simulink model "relay_model_gea_2017a"  (R2019b)
settings: Solver=VariableStepAuto  StartTime=0.0  StopTime=Tsim  RelTol=1e-6
values from neighbouring files (symbols this model uses):
  a1 = x(3)    [relaysim.m]
  a2 = x(2)    [relaysim.m]
  den = sym2poly((s+1)*(0.1*s+1)*(0.01*s+1))    [get_function.m]
  K = x(1)    [relaysim.m]
  num = 1    [get_function.m]
  Td = x(4)    [relaysim.m]
undefined symbols (not defined in the file or in its folder): rd, ri, rp, step_in, Tds
libraries: simulink x1
settings Model: Creator=export08  LastModifiedBy=adrian
settings DataIOCC: ReturnWorkspaceOutputs=off
settings DebuggingCC: ArithmeticOperatorsInVariantConditions=warning
settings SFSimCC: SimUseLocalCustomCode=off  CustomCodeUndefinedFunction=UseInterfaceOnly
settings RTWCC: RTWUseLocalCustomCode=off
settings CodeAppCC: StateflowObjectComments=on

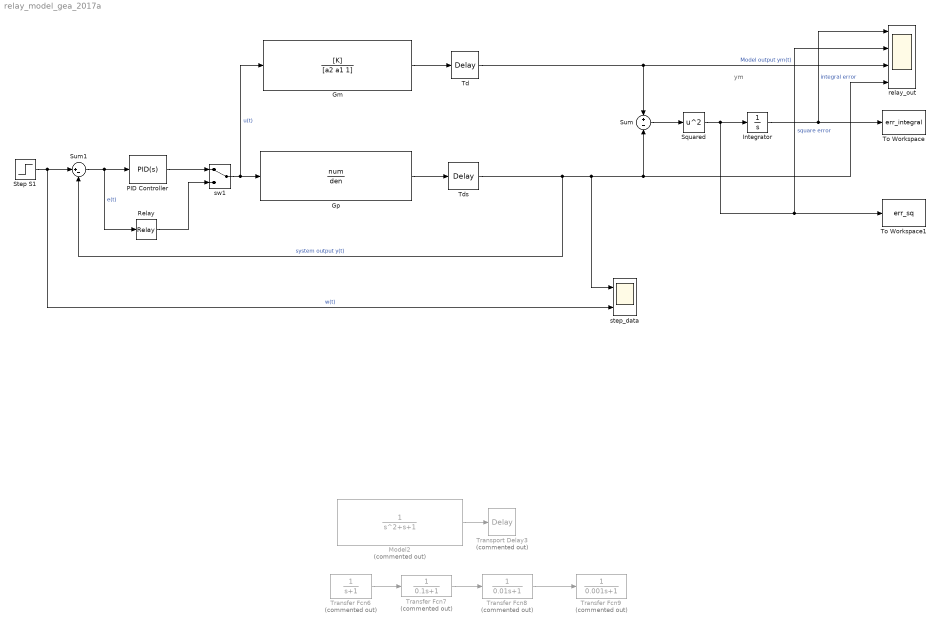
== system relay_model_gea_2017a ==
  note: ym
  Gm : TransferFcn  Numerator=[K]  Denominator=[a2 a1 1]
  Gp : TransferFcn  Numerator=num  Denominator=den
  Integrator : Integrator
  Model2 : TransferFcn  Commented=on  Numerator=1  Denominator=[1 1 1]
  PID Controller : simulink/Continuous/PID Controller  Controller=PID  Form=Parallel  TimeDomain=Continuous-time  SampleTime=-1  IntegratorMethod=Forward Euler  FilterMethod=Forward Euler  ControllerParametersSource=internal  P=rp  I=ri  D=rd  UseFilter=on  N=100  TunerSelectOption=Transfer Function Based (PID Tuner App)  InitialConditionSource=internal  InitialConditionForIntegrator=0  InitialConditionForFilter=0  DifferentiatorICPrevScaledInput=0  ExternalReset=none  TrackingMode=off  Kt=1  LimitOutput=off  UpperSaturationLimit=inf  LowerSaturationLimit=-inf  LinearizeAsGain=on  AntiWindupMode=none  Kb=1  POutMin=[]  POutMax=[]  IOutMin=[]  IOutMax=[]  DOutMin=[]  DOutMax=[]  NOutMin=[]  NOutMax=[]  SumOutMin=[]  SumOutMax=[]  SaturationOutMin=[]  SaturationOutMax=[]  PParamMin=[]  PParamMax=[]  IParamMin=[]  IParamMax=[]  DParamMin=[]  DParamMax=[]  NParamMin=[]  NParamMax=[]  KbParamMin=[]  KbParamMax=[]  KtParamMin=[]  KtParamMax=[]  KbOutMin=[]  KbOutMax=[]  KtOutMin=[]  KtOutMax=[]  IntegratorOutMin=[]  IntegratorOutMax=[]  FilterOutMin=[]  FilterOutMax=[]  SumI1OutMin=[]  SumI1OutMax=[]  SumI2OutMin=[]  SumI2OutMax=[]  SumI3OutMin=[]  SumI3OutMax=[]  SumI4OutMin=[]  SumI4OutMax=[]  SumDOutMin=[]  SumDOutMax=[]  DifferentiatorOutMin=[]  DifferentiatorOutMax=[]  FilterDiffOutCoefMin=[]  FilterDiffOutCoefMax=[]  ReciprocalOutMin=[]  ReciprocalOutMax=[]  SumDenOutMin=[]  SumDenOutMax=[]  SumNumOutMin=[]  SumNumOutMax=[]  DivideOutMin=[]  DivideOutMax=[]  IntegratorContinuousStateAttributes=''  IntegratorStateMustResolveToSignalObject=off  IntegratorRTWStateStorageClass=Auto  FilterContinuousStateAttributes=''  FilterStateMustResolveToSignalObject=off  FilterRTWStateStorageClass=Auto  ParallelPVariant=InternalParameters  IdealPVariant=Disabled  IVariant=InternalParameters  DVariant=InternalParameters  IntegratorVariant=Continuous  SatVariant=Disabled  AWVariant=Passthrough  PCopyVariant=Disabled  TRVariant=Disabled  FdbkBlocksVariant=Forward  IdealPFdbkVariant=Disabled  SatFdbkVariant=Disabled  DerivativeFilterVariant=ContFilter  NVariant=InternalParameters  NCopyVariant=Disabled  FilterICVariant=InternalICsFilter  IntegratorICVariant=InternalICs  ExternalResetVariant=Disabled  TRSumVariant=Passthrough  SumFdbkVariant=Disabled  SumVariant=Sum_PID
  Relay : Relay  OnSwitchValue=0.1  OffSwitchValue=-0.1  OnOutputValue=2  OffOutputValue=-1
  Squared : Math  Operator=square  SaturateOnIntegerOverflow=on
  Step S1 : Step  Time=10  After=step_in  SampleTime=0
  Sum : Sum  Inputs=+-
  Sum1 : Sum  Inputs=|+-
  Td : TransportDelay  DelayTime=Td  BufferSize=5024
  Tds : TransportDelay  DelayTime=Tds
  To Workspace : ToWorkspace  VariableName=err_integral  SaveFormat=Timeseries  SampleTime=-1
  To Workspace1 : ToWorkspace  VariableName=err_sq  SaveFormat=Timeseries  SampleTime=-1
  Transfer Fcn6 : TransferFcn  Commented=on  Denominator=[1 1]
  Transfer Fcn7 : TransferFcn  Commented=on  Denominator=[0.1 1]
  Transfer Fcn8 : TransferFcn  Commented=on  Denominator=[0.01 1]
  Transfer Fcn9 : TransferFcn  Commented=on  Denominator=[0.001 1]
  Transport Delay3 : TransportDelay  Commented=on  BufferSize=5024
  relay_out : Scope  NumInputPorts=4
  step_data : Scope  NumInputPorts=2
  sw1 : ManualSwitch
  wires:
  Gm/1 -> Td/1
  Sum/1 -> Squared/1
  Squared/1 -> Integrator/1, relay_out/2, To Workspace1/1  "square error"
  Integrator/1 -> To Workspace/1, relay_out/1  "integral error"
  Step S1/1 -> step_data/2, Sum1/1  "w(t)"
  Sum1/1 -> Relay/1, PID Controller/1  "e(t)"
  Td/1 -> Sum/1, relay_out/3  "Model output ym(t)"
  PID Controller/1 -> sw1/1
  Model2/1 -> Transport Delay3/1
  Transfer Fcn6/1 -> Transfer Fcn7/1
  Transfer Fcn7/1 -> Transfer Fcn8/1
  Transfer Fcn8/1 -> Transfer Fcn9/1
  Gp/1 -> Tds/1
  Relay/1 -> sw1/2
  sw1/1 -> Gm/1, Gp/1  "u(t)"
  Tds/1 -> step_data/1, Sum/2, relay_out/4, Sum1/2  "system output y(t)"
